simulink model "MIL4L3_SW6_V1_20220211"  (R2018b)
settings: Solver=FixedStepAuto  StartTime=0.0  StopTime=inf  FixedStep=0.001  RelTol=1e-3
PreLoadFcn:
  | A0_MILtest;
undefined symbols (not defined in the file or in its folder): Clb_ICADirect_LaneDisp_StateFive, Clb_ICADirect_LaneDisp_StateFour, Clb_ICADirect_LaneDisp_StateOne, Clb_ICADirect_LaneDisp_StateThree, Clb_ICADirect_LaneDisp_StateTwo, Clb_ICADirect_LaneDisp_StateZero, Clb_ICADirect_LaneDispSW, Clb_ICADirect_TrnLghtsCom_Switch, Clb_ICADirect_TrnLghtsCom_Value, Clb_ICADirect_TrnLghtsCrtl_Inhb, IMAP_Clb_ACU_Driver_Belt, IMAP_Clb_ACU_Driver_Belt_Over, IMAP_Clb_ACU_Passenger_Belt, IMAP_Clb_ACU_Passenger_Belt_Over, IMAP_Clb_ACU_RearLeft_Belt, IMAP_Clb_ACU_RearLeft_Belt_Over, IMAP_Clb_ACU_RearMiddle_Belt, IMAP_Clb_ACU_RearMiddle_Belt_Over, IMAP_Clb_ACU_RearRight_Belt, IMAP_Clb_ACU_RearRight_Belt_Over, IMAP_Clb_AEB_Switch, IMAP_Clb_AEB_Switch_Over, IMAP_Clb_ALC_TLC_Mode, IMAP_Clb_ALC_TLC_Mode_Over, IMAP_Clb_BCM_Battery_Voltage, IMAP_Clb_BCM_Battery_Voltage_Over, IMAP_Clb_BCM_BrakeLamp_State, IMAP_Clb_BCM_BrakeLamp_State_Over, IMAP_Clb_BCM_CHMSL_Status, IMAP_Clb_BCM_CHMSL_Status_Over, IMAP_Clb_BCM_Door_Lock_State, IMAP_Clb_BCM_Door_Lock_State_Over, IMAP_Clb_BCM_FrontWiper_State, IMAP_Clb_BCM_FrontWiper_State_Over, IMAP_Clb_BCM_FrontWiper_Switch, IMAP_Clb_BCM_FrontWiper_Switch_Over, IMAP_Clb_BCM_HazardLamp, IMAP_Clb_BCM_HazardLamp_Over, IMAP_Clb_BCM_HazardLamp_Switch, IMAP_Clb_BCM_HazardLamp_Switch_Over, IMAP_Clb_BCM_HighBeam_State, IMAP_Clb_BCM_HighBeam_State_Over, IMAP_Clb_BCM_Ignition_State, IMAP_Clb_BCM_Ignition_State_Over, IMAP_Clb_BCM_IHBC_Enabled, IMAP_Clb_BCM_IHBC_Enabled_Over, IMAP_Clb_BCM_Left_Light, IMAP_Clb_BCM_Left_Light_Over, IMAP_Clb_BCM_LeftTurn_Switch, IMAP_Clb_BCM_LeftTurn_Switch_Over, IMAP_Clb_BCM_LF_Door_State, IMAP_Clb_BCM_LF_Door_State_Over, IMAP_Clb_BCM_LowBeam_State, IMAP_Clb_BCM_LowBeam_State_Over, IMAP_Clb_BCM_LR_Door_State, IMAP_Clb_BCM_LR_Door_State_Over, IMAP_Clb_BCM_RF_Door_State, IMAP_Clb_BCM_RF_Door_State_Over, IMAP_Clb_BCM_Right_Light, IMAP_Clb_BCM_Right_Light_Over ... (+547)
libraries: CarMaker4SL x2153, simulink x292, dspstat3 x3, canmsglib x2, simulink_extras x1
(part 4 of 52)

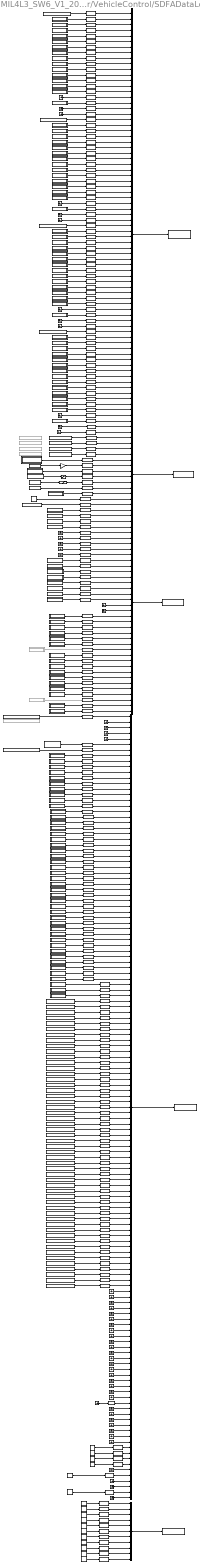
== system MIL4L3_SW6_V1_20220211/CarMaker/VehicleControl/SDFADataLog ==
  ACCEL_LONGI_CALIB2 : Saturate  UpperLimit=40.92  LowerLimit=-40.96
  BusCreator : BusCreator  Inputs=11
  BusCreator1 : BusCreator  Inputs=80
  BusCreator2 : BusCreator  Inputs=40
  BusCreator3 : BusCreator  Inputs=6
  BusCreator4 : BusCreator  Inputs=141
  CIPV_ID1 : Subsystem
  Constant{,1..3,8,10..21} (17 alike) : Constant  Value=0
  Constant9 : Constant
  Data Type  Conversion{1..3,6,508} (5 alike) : DataTypeConversion
  Data Type Conversion{,1..82,85,98,118,128..129,131..251,253..265,267,398,442..444,446..449,451..455} (236 alike) : DataTypeConversion
  Define CM Dict : CarMaker4SL/Define CM Dict  Commented=on  xname=User.IO.Out.CRFLstatus  xmono=off  xtype=Double4  xdvaplace=None  xnstates=0  xfirststate=0  xinitial=0
  Define CM Dict1 : CarMaker4SL/Define CM Dict  Commented=on  xname=User.IO.Out.CRFRstatus  xmono=off  xtype=Double4  xdvaplace=None  xnstates=0  xfirststate=0  xinitial=0
  Define CM Dict3 : CarMaker4SL/Define CM Dict  Commented=on  xname=User.IO.Out.CRRLstatus  xmono=off  xtype=Double4  xdvaplace=None  xnstates=0  xfirststate=0  xinitial=0
  Define CM Dict4 : CarMaker4SL/Define CM Dict  Commented=on  xname=User.IO.Out.CRRRstatus  xmono=off  xtype=Double4  xdvaplace=None  xnstates=0  xfirststate=0  xinitial=0
  Define CM Dict7 : CarMaker4SL/Define CM Dict  Commented=on  xname=User.IO.Out.IFCState  xmono=off  xtype=Double4  xdvaplace=IO_Out  xnstates=0  xfirststate=0  xinitial=9
  Gain10 : Gain  Gain=3.6
  Ground{,1..47,52,56..61} (55 alike) : Ground
  Lateral_acceleration1 : CarMaker4SL/Read CM Dict  xname=Car.ay  xsync=off
  Lateral_acceleration2 : CarMaker4SL/Read CM Dict  xname=User.IO.Out.CRFLstatus  xsync=off
  Lateral_acceleration3 : CarMaker4SL/Read CM Dict  xname=User.IO.Out.CRFRstatus  xsync=off
  Lateral_acceleration4 : CarMaker4SL/Read CM Dict  xname=User.IO.Out.CRRLstatus  xsync=off
  Lateral_acceleration5 : CarMaker4SL/Read CM Dict  xname=User.IO.Out.CRRRstatus  xsync=off
  Read CM Dict : CarMaker4SL/Read CM Dict  xname=User.IO.Out.IFC_Line01_CurvChange  xsync=off
  Read CM Dict1 : CarMaker4SL/Read CM Dict  xname=User.IO.Out.NumberOfObjects_S3  xsync=off
  Read CM Dict10 : CarMaker4SL/Read CM Dict  xname=User.IO.Out.IFC_Line01_Dy  xsync=off
  Read CM Dict11 : CarMaker4SL/Read CM Dict  xname=User.IO.Out.IFC_Line01_ExistProb  xsync=off
  Read CM Dict12 : CarMaker4SL/Read CM Dict  xname=User.IO.Out.IFC_Line01_MeasureType  xsync=off
  Read CM Dict13 : CarMaker4SL/Read CM Dict  xname=User.IO.Out.IFC_Line01_Type  xsync=off
  Read CM Dict14 : CarMaker4SL/Read CM Dict  xname=User.IO.Out.IFC_Line01_LineID  xsync=off
  Read CM Dict15 : CarMaker4SL/Read CM Dict  xname=User.IO.Out.IFC_Line01_TypeConf  xsync=off
  Read CM Dict16 : CarMaker4SL/Read CM Dict  xname=User.IO.Out.IFC_Line01_ColorClass  xsync=off
  Read CM Dict17 : CarMaker4SL/Read CM Dict  xname=User.IO.Out.IFC_Line01_DxStart  xsync=off
  Read CM Dict18 : CarMaker4SL/Read CM Dict  xname=User.IO.Out.IFC_Line01_DxEnd  xsync=off
  Read CM Dict19 : CarMaker4SL/Read CM Dict  xname=User.IO.Out.IFC_Line01_LineWidth  xsync=off
  Read CM Dict2 : CarMaker4SL/Read CM Dict  xname=User.IO.Out.IFCState  xsync=off
  Read CM Dict20 : CarMaker4SL/Read CM Dict  xname=User.IO.Out.IFC_Line02_CurvChange  xsync=off
  Read CM Dict21 : CarMaker4SL/Read CM Dict  xname=User.IO.Out.IFC_Line02_Curv  xsync=off
  Read CM Dict22 : CarMaker4SL/Read CM Dict  xname=User.IO.Out.IFC_Line02_HeadingAngle  xsync=off
  Read CM Dict23 : CarMaker4SL/Read CM Dict  xname=User.IO.Out.IFC_Line02_Dy  xsync=off
  Read CM Dict24 : CarMaker4SL/Read CM Dict  xname=User.IO.Out.IFC_Line02_ExistProb  xsync=off
  Read CM Dict25 : CarMaker4SL/Read CM Dict  xname=Car.ax  xsync=off
  Read CM Dict26 : CarMaker4SL/Read CM Dict  xname=Car.v  xsync=off
  Read CM Dict27 : CarMaker4SL/Read CM Dict  xname=Steer.WhlAng  xsync=off
  Read CM Dict28 : CarMaker4SL/Read CM Dict  xname=User.IO.Out.IFC_Line02_MeasureType  xsync=off
  Read CM Dict29 : CarMaker4SL/Read CM Dict  xname=User.IO.Out.IFC_Line02_Type  xsync=off
  Read CM Dict3 : CarMaker4SL/Read CM Dict  xname=User.IO.Out.NumberOfObjects_S0  xsync=off
  Read CM Dict30 : CarMaker4SL/Read CM Dict  xname=User.IO.Out.IFC_Line02_LineID  xsync=off
  Read CM Dict31 : CarMaker4SL/Read CM Dict  xname=User.IO.Out.IFC_Line02_TypeConf  xsync=off
  Read CM Dict32 : CarMaker4SL/Read CM Dict  xname=User.IO.Out.IFC_Line02_ColorClass  xsync=off
  Read CM Dict33 : CarMaker4SL/Read CM Dict  xname=User.IO.Out.IFC_Line02_DxStart  xsync=off
  Read CM Dict34 : CarMaker4SL/Read CM Dict  xname=User.IO.Out.IFC_Line02_DxEnd  xsync=off
  Read CM Dict35 : CarMaker4SL/Read CM Dict  xname=User.IO.Out.IFC_Line02_LineWidth  xsync=off
  Read CM Dict36 : CarMaker4SL/Read CM Dict  xname=User.IO.Out.IFC_Line03_CurvChange  xsync=off
  Read CM Dict37 : CarMaker4SL/Read CM Dict  xname=User.IO.Out.IFC_Line03_Curv  xsync=off
  Read CM Dict38 : CarMaker4SL/Read CM Dict  xname=User.IO.Out.IFC_Line03_HeadingAngle  xsync=off
  Read CM Dict39 : CarMaker4SL/Read CM Dict  xname=User.IO.Out.IFC_Line03_Dy  xsync=off
  Read CM Dict4 : CarMaker4SL/Read CM Dict  xname=User.IO.Out.NumberOfObjects_S1  xsync=off
  Read CM Dict40 : CarMaker4SL/Read CM Dict  xname=User.IO.Out.IFC_Line03_ExistProb  xsync=off
  Read CM Dict41 : CarMaker4SL/Read CM Dict  xname=User.IO.Out.IFC_Line03_MeasureType  xsync=off
  Read CM Dict42 : CarMaker4SL/Read CM Dict  xname=User.IO.Out.IFC_Line03_Type  xsync=off
  Read CM Dict43 : CarMaker4SL/Read CM Dict  xname=User.IO.Out.IFC_Line03_LineID  xsync=off
  Read CM Dict44 : CarMaker4SL/Read CM Dict  xname=User.IO.Out.IFC_Line03_TypeConf  xsync=off
  Read CM Dict45 : CarMaker4SL/Read CM Dict  xname=User.IO.Out.IFC_Line03_ColorClass  xsync=off
  Read CM Dict46 : CarMaker4SL/Read CM Dict  xname=User.IO.Out.IFC_Line03_DxStart  xsync=off
  Read CM Dict47 : CarMaker4SL/Read CM Dict  xname=User.IO.Out.IFC_Line03_DxEnd  xsync=off
  Read CM Dict48 : CarMaker4SL/Read CM Dict  xname=User.IO.Out.IFC_Line03_LineWidth  xsync=off
  Read CM Dict49 : CarMaker4SL/Read CM Dict  xname=User.IO.Out.IFC_Line04_CurvChange  xsync=off
  Read CM Dict5 : CarMaker4SL/Read CM Dict  xname=User.IO.Out.NumberOfObjects_S2  xsync=off
  Read CM Dict50 : CarMaker4SL/Read CM Dict  xname=User.IO.Out.IFC_Line04_Curv  xsync=off
  Read CM Dict51 : CarMaker4SL/Read CM Dict  xname=User.IO.Out.IFC_Line04_HeadingAngle  xsync=off
  Read CM Dict52 : CarMaker4SL/Read CM Dict  xname=User.IO.Out.IFC_Line04_Dy  xsync=off
  Read CM Dict53 : CarMaker4SL/Read CM Dict  xname=User.IO.Out.IFC_Line04_ExistProb  xsync=off
  Read CM Dict54 : CarMaker4SL/Read CM Dict  xname=User.IO.Out.IFC_Line04_MeasureType  xsync=off
  Read CM Dict55 : CarMaker4SL/Read CM Dict  xname=User.IO.Out.IFC_Line04_Type  xsync=off
  Read CM Dict56 : CarMaker4SL/Read CM Dict  xname=User.IO.Out.IFC_Line04_LineID  xsync=off
  Read CM Dict57 : CarMaker4SL/Read CM Dict  xname=User.IO.Out.IFC_Line04_TypeConf  xsync=off
  Read CM Dict58 : CarMaker4SL/Read CM Dict  xname=User.IO.Out.IFC_Line04_ColorClass  xsync=off
  Read CM Dict59 : CarMaker4SL/Read CM Dict  xname=User.IO.Out.IFC_Line04_DxStart  xsync=off
  Read CM Dict6 : CarMaker4SL/Read CM Dict  xname=User.IO.Out.NumberOfObj  xsync=off
  Read CM Dict60 : CarMaker4SL/Read CM Dict  xname=User.IO.Out.IFC_Line04_DxEnd  xsync=off
  Read CM Dict61 : CarMaker4SL/Read CM Dict  xname=User.IO.Out.IFC_Line04_LineWidth  xsync=off
  Read CM Dict62 : CarMaker4SL/Read CM Dict  xname=User.IO.Out.ObjCount  xsync=off
  Read CM Dict8 : CarMaker4SL/Read CM Dict  xname=User.IO.Out.IFC_Line01_Curv  xsync=off
  Read CM Dict9 : CarMaker4SL/Read CM Dict  xname=User.IO.Out.IFC_Line01_HeadingAngle  xsync=off
  Saturation3 : Saturate  UpperLimit=780  LowerLimit=-780
  Subsystem : Subsystem
  Subsystem1 : Subsystem
  Subsystem10 : Subsystem
  Subsystem100 : Subsystem
  Subsystem103 : Subsystem
  Subsystem107 : Subsystem
  Subsystem108 : Subsystem
  Subsystem109 : Subsystem
  Subsystem11 : Subsystem
  Subsystem110 : Subsystem
  Subsystem111 : Subsystem
  Subsystem112 : Subsystem
  Subsystem113 : Subsystem
  Subsystem114 : Subsystem
  Subsystem115 : Subsystem
  Subsystem116 : Subsystem
  Subsystem117 : Subsystem
  Subsystem118 : Subsystem
  Subsystem119 : Subsystem
  Subsystem12 : Subsystem
  Subsystem120 : Subsystem
  Subsystem13 : Subsystem  Commented=on
  Subsystem14 : Subsystem
  Subsystem149 : Subsystem
  Subsystem150 : Subsystem
  Subsystem160 : Subsystem
  Subsystem171 : Subsystem
  Subsystem174 : Subsystem
  Subsystem175 : Subsystem
  Subsystem176 : Subsystem
  Subsystem177 : Subsystem
  Subsystem178 : Subsystem
  Subsystem179 : Subsystem
  Subsystem180 : Subsystem
  Subsystem181 : Subsystem
  Subsystem182 : Subsystem
  Subsystem183 : Subsystem
  Subsystem184 : Subsystem
  Subsystem185 : Subsystem
  Subsystem186 : Subsystem
  Subsystem187 : Subsystem
  Subsystem188 : Subsystem
  Subsystem189 : Subsystem
  Subsystem190 : Subsystem
  Subsystem191 : Subsystem
  Subsystem192 : Subsystem
  Subsystem193 : Subsystem
  Subsystem194 : Subsystem
  Subsystem195 : Subsystem
  Subsystem196 : Subsystem
  Subsystem197 : Subsystem
  Subsystem198 : Subsystem
  Subsystem199 : Subsystem
  Subsystem2 : Subsystem
  Subsystem20 : Subsystem
  Subsystem200 : Subsystem
  Subsystem201 : Subsystem
  Subsystem202 : Subsystem
  Subsystem203 : Subsystem
  Subsystem204 : Subsystem
  Subsystem205 : Subsystem
  Subsystem206 : Subsystem
  Subsystem208 : Subsystem
  Subsystem209 : Subsystem
  Subsystem210 : Subsystem
  Subsystem211 : Subsystem
  Subsystem212 : Subsystem
  Subsystem213 : Subsystem  Commented=on
  Subsystem214 : Subsystem
  Subsystem215 : Subsystem
  Subsystem216 : Subsystem
  Subsystem217 : Subsystem
  Subsystem218 : Subsystem
  Subsystem219 : Subsystem
  Subsystem220 : Subsystem
  Subsystem221 : Subsystem
  Subsystem222 : Subsystem
  Subsystem223 : Subsystem
  Subsystem224 : Subsystem
  Subsystem225 : Subsystem
  Subsystem226 : Subsystem
  Subsystem227 : Subsystem
  Subsystem228 : Subsystem
  Subsystem232 : Subsystem
  Subsystem255 : Subsystem
  Subsystem283 : Subsystem
  Subsystem3 : Subsystem
  Subsystem40 : Subsystem
  Subsystem46 : Subsystem
  Subsystem47 : Subsystem
  Subsystem48 : Subsystem
  Subsystem49 : Subsystem
  Subsystem5 : Subsystem
  Subsystem50 : Subsystem
  Subsystem51 : Subsystem
  Subsystem52 : Subsystem
  Subsystem53 : Subsystem
  Subsystem54 : Subsystem
  Subsystem55 : Subsystem
  Subsystem56 : Subsystem
  Subsystem57 : Subsystem
  Subsystem58 : Subsystem
  Subsystem59 : Subsystem
  Subsystem6 : Subsystem
  Subsystem61 : Subsystem
  Subsystem66 : Subsystem
  Subsystem67 : Subsystem
  Subsystem68 : Subsystem
  Subsystem69 : Subsystem
  Subsystem7 : Subsystem
  Subsystem70 : Subsystem
  Subsystem71 : Subsystem
  Subsystem72 : Subsystem
  Subsystem73 : Subsystem
  Subsystem74 : Subsystem
  Subsystem75 : Subsystem
  Subsystem76 : Subsystem
  Subsystem77 : Subsystem
  Subsystem78 : Subsystem
  Subsystem79 : Subsystem
  Subsystem8 : Subsystem
  Subsystem81 : Subsystem
  Subsystem85 : Subsystem
  Subsystem86 : Subsystem
  Subsystem87 : Subsystem
  Subsystem88 : Subsystem
  Subsystem89 : Subsystem
  Subsystem9 : Subsystem
  Subsystem90 : Subsystem
  Subsystem91 : Subsystem
  Subsystem92 : Subsystem
  Subsystem93 : Subsystem
  Subsystem94 : Subsystem
  Subsystem95 : Subsystem
  Subsystem96 : Subsystem
  Subsystem97 : Subsystem
  Subsystem98 : Subsystem
  To Workspace : ToWorkspace  VariableName=CameraDataLog  SaveFormat=Timeseries  SampleTime=-1
  To Workspace1 : ToWorkspace  VariableName=RadarDataLog  SaveFormat=Timeseries  SampleTime=-1
  To Workspace2 : ToWorkspace  VariableName=VehicleDataLog  SaveFormat=Timeseries  SampleTime=-1
  To Workspace3 : ToWorkspace  VariableName=CRDataLog  SaveFormat=Timeseries  SampleTime=-1
  To Workspace4 : ToWorkspace  VariableName=LAPDataLog  SaveFormat=Timeseries  SampleTime=-1
  wires:
  BusCreator3/1 -> To Workspace2/1  "VehicleData"
  BusCreator4/1 -> To Workspace/1  "CameraData"
  BusCreator2/1 -> To Workspace1/1  "RadarData"
  BusCreator1/1 -> To Workspace3/1  "CRData"
  Subsystem13/1(BrakingAllowed) -> Data Type Conversion82/1
  Data Type Conversion232/1 -> BusCreator4/86  "LH_Lanemark_Type_Conf_03"
  Subsystem6/1(obj_HeadOrientation) -> Data Type Conversion74/1
  Data Type Conversion70/1 -> BusCreator2/32  "ObjectAge"
  Data Type Conversion/1 -> BusCreator4/132  "CorrCoeff_x_vx"
  Data Type Conversion215/1 -> BusCreator4/70  "IFC_Line02_MeasureType"
  Data Type Conversion27/1 -> BusCreator4/20  "IFC_obj_abs_AxStdDev"
  Data Type Conversion235/1 -> BusCreator4/12  "IFC_obj_VxValid"
  Data Type Conversion249/1 -> BusCreator4/101  "IFC_Line04_DxStart"
  Data Type Conversion59/1 -> BusCreator4/57  "IFC_Line01_MeasureType"
  Read CM Dict34/1 -> Data Type Conversion221/1
  Read CM Dict36/1 -> Data Type Conversion223/1
  Subsystem10/1(obj_PhiBottom) -> Data Type Conversion78/1
  Subsystem7/1(obj_DirIndicator) -> Data Type Conversion75/1
  Data Type Conversion261/1 -> BusCreator2/9  "RelativeLongVelo"
  Subsystem198/1(obj_Rel_VxSTD) -> Data Type Conversion29/1
  Data Type Conversion58/1 -> BusCreator4/56  "IFC_Line01_ExistProb"
  Data Type Conversion260/1 -> BusCreator2/10  "RelativeLatVelo"
  Data Type Conversion57/1 -> BusCreator4/55  "IFC_Line01_Dy"
  Data Type Conversion213/1 -> BusCreator4/8  "IFC_obj_ExistProb"
  Data Type Conversion197/1 -> BusCreator1/63  "RBtar_Yvelocity"
  Data Type Conversion74/1 -> BusCreator4/47  "IFC_obj_HeadOrientation"
  Subsystem191/1(obj_PhiBottomSTD) -> Data Type Conversion22/1
  Data Type Conversion51/1 -> BusCreator4/49  "IFC_obj_TTIPC"
  Data Type Conversion205/1 -> BusCreator1/70  "RBtar_Class"
  Read CM Dict10/1 -> Data Type Conversion57/1
  Gain10/1 -> Data Type  Conversion508/1  "Vehicle_speed_of_wheelsensor"
  Subsystem193/1(obj_DxSTD) -> Data Type Conversion24/1
  Read CM Dict48/1 -> Data Type Conversion237/1
  Data Type Conversion150/1 -> BusCreator1/13  "LFtar_Class"
  Subsystem20/1(Yaw_speed) -> Data Type  Conversion1/1  "Yaw_speed"
  Ground/1 -> BusCreator4/136  "IsNew"
  Subsystem180/1(WidhSTD) -> Data Type Conversion11/1
  Constant1/1 -> Data Type Conversion118/1
  Data Type Conversion129/1 -> BusCreator4/135  "CorrCoeff_x_vy"
  Data Type Conversion224/1 -> BusCreator4/11  "IFC_obj_Rel_Vx"
  Subsystem216/1(obj_Width) -> Data Type Conversion44/1
  Data Type Conversion194/1 -> BusCreator1/60  "RBtar_Xpos"
  Data Type Conversion195/1 -> BusCreator1/62  "RBtar_Xvelocity"
  Read CM Dict47/1 -> Data Type Conversion236/1
  Data Type Conversion53/1 -> BusCreator4/52  "IFC_Line01_CurvChange"
  Data Type Conversion151/1 -> BusCreator1/14  "LFtar_ReferencePoint"
  Data Type Conversion247/1 -> BusCreator4/99  "LH_Lanemark_Type_Conf_04"
  Read CM Dict26/1 -> Gain10/1
  Subsystem196/1(obj_abs_AxSTD) -> Data Type Conversion27/1
  Data Type Conversion118/1 -> BusCreator4/133  "CorrCoeff_y_vy"
  Constant/1 -> Data Type Conversion/1
  Data Type  Conversion1/1 -> BusCreator3/3  "SWINve_g_ESC_YawRate"
  Read CM Dict20/1 -> Data Type Conversion67/1
  Subsystem9/1(obj_angle_3D) -> Data Type Conversion77/1
  Data Type Conversion65/1 -> BusCreator4/63  "IFC_Line01_DxEnd"
  Read CM Dict53/1 -> Data Type Conversion242/1
  Read CM Dict18/1 -> Data Type Conversion65/1
  Read CM Dict46/1 -> Data Type Conversion234/1
  Read CM Dict60/1 -> Data Type Conversion250/1
  Subsystem201/1(AbsoluteLatAcc) -> Data Type Conversion255/1
  Data Type Conversion30/1 -> BusCreator4/17  "IFC_obj_Rel_VyStdDev"
  Ground34/1 -> BusCreator4/127  "FS_Blur_Image_0"
  Subsystem150/1(AbsoluteLongAcc) -> Data Type Conversion258/1
  Subsystem199/1(obj_Rel_VySTD) -> Data Type Conversion30/1
  Subsystem204/1(obj_abs_Ay) -> Data Type Conversion33/1
  Ground52/1 -> Data Type Conversion72/1
  Data Type Conversion241/1 -> BusCreator4/94  "IFC_Line04_Dy"
  Data Type Conversion254/1 -> BusCreator2/23  "ClassType"
  Subsystem228/1(obj_Type) -> Data Type Conversion50/1
  Subsystem78/1(RFtar_ReferencePoint) -> Data Type Conversion168/1  "RFtar_ReferencePoint"
  Ground25/1 -> BusCreator4/123  "IFC_Roaddge02_LineID"
  Data Type Conversion147/1 -> BusCreator1/10  "LFtar_Length"
  Data Type Conversion85/1 -> BusCreator3/1  "system_clock"
  Data Type Conversion133/1 -> BusCreator1/79
  Read CM Dict28/1 -> Data Type Conversion215/1
  Data Type  Conversion6/1 -> BusCreator3/5  "SWINve_g_ESC_LongitudinalAccelaration"
  Subsystem227/1(obj_Measured) -> Data Type Conversion52/1
  Data Type Conversion239/1 -> BusCreator4/92  "IFC_Line04_Curv"
  Subsystem160/1(obj_Rel_Vx) -> Data Type Conversion224/1
  Read CM Dict43/1 -> Data Type Conversion231/1
  Subsystem195/1(obj_PhiLeftSTD) -> Data Type Conversion26/1
  Data Type Conversion5/1 -> BusCreator2/7  "LateralDistanceSTD"
  Read CM Dict32/1 -> Data Type Conversion219/1
  Read CM Dict27/1 -> Saturation3/1  "Steering_wheel_angle"
  Subsystem232/1(ClassProbValue) -> Data Type Conversion253/1
  Data Type Conversion75/1 -> BusCreator4/44  "IFC_obj_DirIndicator"
  Read CM Dict42/1 -> Data Type Conversion230/1
  Data Type  Conversion2/1 -> BusCreator3/4  "SWINve_g_SAS_SteeringAngle"
  Ground3/1 -> Data Type Conversion261/1
  Subsystem76/1(RFtar_ExistenceProbability) -> Data Type Conversion166/1  "RFtar_ExistenceProbability"
  Subsystem174/1(LateralDistanceSTD) -> Data Type Conversion5/1
  Subsystem118/1(RBtar_Class) -> Data Type Conversion205/1  "RBtar_Class"
  Read CM Dict35/1 -> Data Type Conversion222/1
  Ground39/1 -> BusCreator4/131  "FS_Out_Of_Focus_0"
  Data Type Conversion220/1 -> BusCreator4/75  "IFC_Line02_DxStart"
  Read CM Dict23/1 -> Data Type Conversion212/1
  Ground57/1 -> BusCreator4/3  "FS_Sun_Ray_0"
  Data Type Conversion227/1 -> BusCreator4/81  "IFC_Line03_Dy"
  Read CM Dict33/1 -> Data Type Conversion220/1
  Subsystem175/1(LongDistanceSTD) -> Data Type Conversion4/1
  Subsystem52/1(LFtar_Yacceleration) -> Data Type Conversion145/1  "LFtar_Yacceleration"
  Ground9/1 -> Data Type Conversion263/1
  Subsystem213/1(Height) -> Data Type Conversion42/1
  Subsystem176/1(AbsoluteLongAccSTD) -> Data Type Conversion7/1
  Data Type Conversion18/1 -> BusCreator4/40  "IFC_obj_HeightStdDev"
  Ground61/1 -> BusCreator2/22  "AbsAccCov"
  Data Type Conversion221/1 -> BusCreator4/76  "IFC_Line02_DxEnd"
  Subsystem149/1(obj_ExistProb) -> Data Type Conversion213/1
  Subsystem219/1(YawAngle) -> Data Type Conversion36/1
  Data Type Conversion258/1 -> BusCreator2/15  "AbsoluteLongAcc"
  Data Type Conversion46/1 -> BusCreator2/25  "Length"
  Subsystem1/1(LongDistance) -> Data Type Conversion267/1
  Read CM Dict59/1 -> Data Type Conversion249/1
  Data Type Conversion211/1 -> BusCreator4/67  "IFC_Line02_HeadingAngle"
  Data Type Conversion226/1 -> BusCreator4/80  "IFC_Line03_HeadingAngle"
  Data Type Conversion257/1 -> BusCreator2/40  "ExistenceProb"
  Read CM Dict9/1 -> Data Type Conversion55/1
  Subsystem107/1(RBtar_id) -> Data Type Conversion192/1  "RBtar_id"
  Subsystem221/1(MovementStatus) -> Data Type Conversion34/1
  Data Type Conversion216/1 -> BusCreator4/71  "IFC_Line02_Type"
  Read CM Dict52/1 -> Data Type Conversion241/1
  Data Type Conversion8/1 -> BusCreator2/18  "AbsLatVeloSTD"
  Read CM Dict13/1 -> Data Type Conversion61/1
  Data Type Conversion12/1 -> BusCreator2/30  "HeightSTD"
  Read CM Dict58/1 -> Data Type Conversion248/1
  Read CM Dict50/1 -> Data Type Conversion239/1
  Subsystem189/1(obj_HeadingSTD) -> Data Type Conversion20/1
  Subsystem209/1(Length) -> Data Type Conversion46/1
  Subsystem66/1(RFtar_id) -> Data Type Conversion154/1  "RFtar_id"
  Data Type Conversion33/1 -> BusCreator4/21  "IFC_obj_abs_Ay"
  Subsystem90/1(LBtar_Xacceleration) -> Data Type Conversion179/1  "LBtar_Xacceleration"
  Read CM Dict16/1 -> Data Type Conversion63/1
  Data Type Conversion191/1 -> BusCreator1/58  "RBtar_number"
  Read CM Dict17/1 -> Data Type Conversion64/1
  Data Type Conversion217/1 -> BusCreator4/72  "IFC_Line02_LineID"
  Data Type Conversion24/1 -> BusCreator4/24  "IFC_obj_DxStdDev"
  Data Type  Conversion3/1 -> BusCreator3/6  "SWINve_g_ESC_LateralAccelaration"
  Subsystem192/1(obj_Rel_Vy) -> Data Type Conversion246/1
  Ground18/1 -> Data Type Conversion206/1  "RBtar_ObjectInfo"
  Ground31/1 -> BusCreator4/117  "IFC_Roaddge02_Curv"
  Read CM Dict57/1 -> Data Type Conversion247/1
  Subsystem222/1(MeasurementStatus) -> Data Type Conversion32/1
  Data Type Conversion264/1 -> BusCreator2/3  "NumberOfObj"
  Read CM Dict3/1 -> Data Type Conversion172/1  "LBtar_number"
  ACCEL_LONGI_CALIB2/1 -> Data Type  Conversion6/1  "ACCEL_LONGI_CALIB"
  Subsystem203/1(obj_abs_Ax) -> Data Type Conversion23/1
  Read CM Dict45/1 -> Data Type Conversion233/1
  Data Type Conversion253/1 -> BusCreator2/24  "ClassProbValue"
  Data Type Conversion156/1 -> BusCreator1/23  "RFtar_Ypos"
  Data Type Conversion256/1 -> BusCreator2/17  "AbsoluteLatVelo"
  Subsystem214/1(obj_PhiRight) -> Data Type Conversion41/1
  Data Type Conversion52/1 -> BusCreator4/51  "IFC_obj_Measured"
  Ground26/1 -> BusCreator4/113  "IFC_Roaddge01_LineID"
  Data Type Conversion66/1 -> BusCreator4/64  "IFC_Line01_LineWidth"
  Subsystem255/1(AbsoluteLongVeloSTD) -> Data Type Conversion6/1
  Subsystem55/1(LFtar_Orientation) -> Data Type Conversion148/1  "LFtar_Orientation"
  Read CM Dict8/1 -> Data Type Conversion54/1
  Data Type Conversion42/1 -> BusCreator2/29  "Height"
  Data Type Conversion16/1 -> BusCreator4/38  "IFC_obj_WidthStdDev"
  Data Type Conversion20/1 -> BusCreator4/46  "IFC_obj_HeadingStdDev"
  Data Type Conversion233/1 -> BusCreator4/87  "IFC_Line03_ColorClass"
  Data Type Conversion225/1 -> BusCreator4/79  "IFC_Line03_Curv"
  Data Type Conversion41/1 -> BusCreator4/29  "IFC_obj_PhiRight"
  Data Type Conversion63/1 -> BusCreator4/61  "IFC_Line01_ColorClass"
  Ground58/1 -> BusCreator4/4  "FS_Fog"
  Data Type Conversion37/1 -> BusCreator4/25  "IFC_obj_Dy"
  Ground17/1 -> Data Type Conversion152/1  "LFtar_timestamp"
  Subsystem119/1(RBtar_ReferencePoint) -> Data Type Conversion204/1  "RBtar_ReferencePoint"
  Data Type Conversion243/1 -> BusCreator4/96  "IFC_Line04_MeasureType"
  Data Type Conversion49/1 -> BusCreator4/45  "IFC_obj_Heading"
  Data Type Conversion265/1 -> BusCreator2/2  "ObjectListQuali"
  Data Type Conversion55/1 -> BusCreator4/54  "IFC_Line01_HeadingAngle"
  Data Type Conversion40/1 -> BusCreator2/31  "ObjectID"
  Subsystem177/1(AbsoluteLatVeloSTD) -> Data Type Conversion8/1
  Read CM Dict39/1 -> Data Type Conversion227/1
  Subsystem188/1(obj_LengthSTD) -> Data Type Conversion19/1
  Subsystem200/1(obj_abgle_3DSTD) -> Data Type Conversion31/1
  Saturation3/1 -> Data Type  Conversion2/1
  Data Type Conversion76/1 -> BusCreator4/35  "IFC_obj_angle_rate"
  Ground38/1 -> Data Type Conversion169/1  "RFtar_ObjectInfo"
  Data Type Conversion244/1 -> BusCreator4/97  "IFC_Line04_Type"
  Data Type Conversion248/1 -> BusCreator4/100  "IFC_Line04_ColorClass"
  Data Type Conversion29/1 -> BusCreator4/15  "IFC_obj_Rel_VxStdDev"
  Ground40/1 -> Data Type Conversion171/1  "RFtar_timestamp"
  Read CM Dict11/1 -> Data Type Conversion58/1
  Subsystem187/1(obj_HeightSTD) -> Data Type Conversion18/1
  Data Type Conversion10/1 -> BusCreator2/26  "LengthSTD"
  Ground28/1 -> BusCreator4/115  "IFC_Roaddge02_MessureType"
  Subsystem205/1(ClassType) -> Data Type Conversion254/1
  Read CM Dict5/1 -> Data Type Conversion138/1
  Data Type  Conversion508/1 -> BusCreator3/2  "SWINve_g_ESC_VeSpd"
  Subsystem224/1(obj_Heading) -> Data Type Conversion49/1
  Data Type Conversion1/1 -> BusCreator4/9  "IFC_obj_TypePron"
  Data Type Conversion181/1 -> BusCreator1/47  "LBtar_Width"
  Lateral_acceleration2/1 -> Data Type Conversion131/1
  Data Type Conversion155/1 -> BusCreator1/22  "RFtar_Xpos"
  Data Type Conversion171/1 -> BusCreator1/38  "RFtar_timestamp"
  Subsystem212/1(obj_PhiLeft) -> Data Type Conversion38/1
  Data Type Conversion79/1 -> BusCreator4/18  "IFC_obj_Rel_VyStdDevValid"
  Data Type Conversion21/1 -> BusCreator4/50  "IFC_obj_TTIPC_StdDev"
  Data Type Conversion238/1 -> BusCreator4/91  "IFC_Line04_CurvChange"
  Ground10/1 -> BusCreator4/108  "IFC_Roaddge01_HeadingAngle"
  Data Type Conversion31/1 -> BusCreator4/34  "IFC_obj_angle_3DStdDev"
  Ground56/1 -> BusCreator4/2  "FS_Low_Sun_0"
  Subsystem49/1(LFtar_Xvelocity) -> Data Type Conversion142/1  "LFtar_Xvelocity"
  Subsystem85/1(LBtar_id) -> Data Type Conversion173/1  "LBtar_id"
  Subsystem215/1(ObjectID) -> Data Type Conversion40/1
  Subsystem182/1(AbsoluteLatVelo) -> Data Type Conversion256/1
  Data Type Conversion7/1 -> BusCreator2/16  "AbsoluteLongAccSTD"
  Data Type Conversion28/1 -> BusCreator4/22  "IFC_obj_abs_AyStdDev"
  Read CM Dict15/1 -> Data Type Conversion62/1
  Subsystem202/1(obj_Rel_VyValid) -> Data Type Conversion2/1
  Data Type Conversion14/1 -> BusCreator2/35  "YawSTD"
  Data Type Conversion15/1 -> BusCreator4/30  "IFC_obj_PhiRightStdDev"
  Read CM Dict25/1 -> ACCEL_LONGI_CALIB2/1
  Data Type Conversion3/1 -> BusCreator2/6  "LatDistance"
  Ground21/1 -> BusCreator4/119  "IFC_Roaddge02_Dy"
  Read CM Dict21/1 -> Data Type Conversion68/1
  Read CM Dict38/1 -> Data Type Conversion226/1
  CIPV_ID1/1(Out1) -> Data Type Conversion39/1  "CIVP_ID"
  Ground19/1 -> BusCreator4/118  "IFC_Roaddge02_HeadingAngle"
  Data Type Conversion22/1 -> BusCreator4/32  "IFC_obj_PhiBottomStdDev"
  Data Type Conversion36/1 -> BusCreator2/34  "YawAngle"
  Ground16/1 -> BusCreator4/112  "IFC_Roaddge01_ExistProb"
  Data Type Conversion35/1 -> BusCreator4/23  "IFC_obj_Dx"
  Constant2/1 -> Data Type Conversion128/1
  Data Type Conversion186/1 -> BusCreator1/51  "LBtar_Class"
  Data Type Conversion43/1 -> BusCreator2/27  "Widh"
  Data Type Conversion38/1 -> BusCreator4/27  "IFC_obj_PhiLeft"
  Ground27/1 -> BusCreator4/114  "IFC_Roaddge02_Type"
  Data Type Conversion34/1 -> BusCreator2/36  "MovementStatus"
  Read CM Dict30/1 -> Data Type Conversion217/1
  Ground24/1 -> BusCreator4/121  "IFC_Roaddge02_DxStart"
  Ground30/1 -> BusCreator4/116  "IFC_Roaddge02_CurvChange"
  Ground2/1 -> BusCreator4/122  "IFC_Roaddge02_ExistProb"
  Data Type Conversion219/1 -> BusCreator4/74  "IFC_Line02_ColorClass"
  Data Type Conversion78/1 -> BusCreator4/31  "IFC_obj_PhiBottom"
  Subsystem184/1(obj_PhiRightSTD) -> Data Type Conversion15/1
  Data Type Conversion230/1 -> BusCreator4/84  "IFC_Line03_Type"
  Subsystem11/1(obj_Rel_VyStdDevValid) -> Data Type Conversion79/1
  Ground33/1 -> BusCreator4/126  "FS_Splashes_0"
  Ground7/1 -> BusCreator4/107  "IFC_Roaddge01_Curv"
  Data Type Conversion73/1 -> BusCreator4/48  "IFC_obj_BrakeLight"
  Read CM Dict19/1 -> Data Type Conversion66/1
  Ground23/1 -> BusCreator4/120  "IFC_Roaddge02_DxEnd"
  Read CM Dict61/1 -> Data Type Conversion251/1
  Subsystem12/1(obj_Rel_VxStdDevValid) -> Data Type Conversion80/1
  Subsystem97/1(LBtar_ReferencePoint) -> Data Type Conversion187/1  "LBtar_ReferencePoint"
  Data Type Conversion11/1 -> BusCreator2/28  "WidhSTD"
  Ground14/1 -> Data Type Conversion158/1  "LFtar_ObjectInfo"
  Subsystem103/1(RBtar_ClassHighestProb) -> Data Type Conversion208/1  "RBtar_ClassHighestProb"
  Data Type Conversion141/1 -> BusCreator1/4  "LFtar_Ypos"
  Subsystem95/1(LBtar_ExistenceProbability) -> Data Type Conversion184/1  "LBtar_ExistenceProbability"
  Subsystem206/1(Latdistance) -> Data Type Conversion3/1
  Data Type Conversion61/1 -> BusCreator4/58  "IFC_Line01_Type"
  Read CM Dict40/1 -> Data Type Conversion228/1
  Data Type Conversion174/1 -> BusCreator1/18  "LFtar_MessageCounter"
  Data Type Conversion183/1 -> BusCreator1/49  "LBtar_Orientation"
  Subsystem57/1(LFtar_Class) -> Data Type Conversion150/1  "LFtar_Class"
  Subsystem120/1(RBtar_MovingState) -> Data Type Conversion136/1
  Data Type Conversion229/1 -> BusCreator4/83  "IFC_Line03_MeasureType"
  Subsystem54/1(LFtar_Length) -> Data Type Conversion147/1  "LFtar_Length"
  Ground15/1 -> Data Type Conversion174/1
  Subsystem194/1(obj_DySTD) -> Data Type Conversion25/1
  Ground37/1 -> BusCreator4/130  "FS_Full_Windshield_0"
  Subsystem59/1(LFtar_MovingState) -> Data Type Conversion185/1
  Data Type Conversion209/1 -> BusCreator1/76  "RBtar_timestamp"
  Subsystem111/1(RBtar_Yvelocity) -> Data Type Conversion197/1  "RBtar_Yvelocity"
  Subsystem77/1(RFtar_Class) -> Data Type Conversion167/1  "RFtar_Class"
  Data Type Conversion131/1 -> BusCreator1/77
  Subsystem88/1(LBtar_Xvelocity) -> Data Type Conversion177/1  "LBtar_Xvelocity"
  Read CM Dict37/1 -> Data Type Conversion225/1
  Ground22/1 -> Data Type Conversion188/1  "LBtar_ObjectInfo"
  Data Type Conversion67/1 -> BusCreator4/65  "IFC_Line02_CurvChange"
  Data Type Conversion132/1 -> BusCreator1/78
  Data Type Conversion64/1 -> BusCreator4/62  "IFC_Line01_DxStart"
  Subsystem115/1(RBtar_Length) -> Data Type Conversion201/1  "RBtar_Length"
  Subsystem81/1(RFtar_ClassHighestProb) -> Data Type Conversion170/1  "RFtar_ClassHighestProb"
  Data Type Conversion152/1 -> BusCreator1/19  "LFtar_timestamp"
  Subsystem108/1(RBtar_Xpos) -> Data Type Conversion194/1  "RBtar_Xpos"
  Subsystem114/1(RBtar_Width) -> Data Type Conversion199/1  "RBtar_Width"
  Data Type Conversion207/1 -> BusCreator1/37  "RFtar_MessageCounter"
  Subsystem110/1(RBtar_Xvelocity) -> Data Type Conversion195/1  "RBtar_Xvelocity"
  Subsystem113/1(RBtar_Yacceleration) -> Data Type Conversion200/1  "RBtar_Yacceleration"
  Read CM Dict44/1 -> Data Type Conversion232/1
  Subsystem72/1(RFtar_Yacceleration) -> Data Type Conversion162/1  "RFtar_Yacceleration"
  Data Type Conversion145/1 -> BusCreator1/8  "LFtar_Yacceleration"
  Ground45/1 -> Data Type Conversion135/1
  Subsystem50/1(LFtar_Yvelocity) -> Data Type Conversion143/1  "LFtar_Yvelocity"
  Data Type Conversion77/1 -> BusCreator4/33  "IFC_obj_angle_3D"
  Data Type Conversion153/1 -> BusCreator1/20  "RFtar_number"
  Data Type Conversion68/1 -> BusCreator4/66  "IFC_Line02_Curv"
  Data Type Conversion164/1 -> BusCreator1/29  "RFtar_Length"
  Ground41/1 -> Data Type Conversion207/1
  Subsystem58/1(LFtar_ReferencePoint) -> Data Type Conversion151/1  "LFtar_ReferencePoint"
  Subsystem96/1(LBtar_Class) -> Data Type Conversion186/1  "LBtar_Class"
  Data Type Conversion176/1 -> BusCreator1/42  "LBtar_Ypos"
  Data Type Conversion17/1 -> BusCreator4/36  "IFC_obj_angle_rate_StdDev"
  Subsystem87/1(LBtar_Ypos) -> Data Type Conversion176/1  "LBtar_Ypos"
  Subsystem69/1(RFtar_Xvelocity) -> Data Type Conversion157/1  "RFtar_Xvelocity"
  Data Type Conversion13/1 -> BusCreator4/1  "IFC_State"
  Subsystem74/1(RFtar_Length) -> Data Type Conversion164/1  "RFtar_Length"
  Subsystem100/1(LBtar_ClassHighestProb) -> Data Type Conversion189/1  "LBtar_ClassHighestProb"
  Subsystem68/1(RFtar_Ypos) -> Data Type Conversion156/1  "RFtar_Ypos"
  Data Type Conversion204/1 -> BusCreator1/71  "RBtar_ReferencePoint"
  Ground42/1 -> Data Type Conversion69/1
  Subsystem218/1(obj_Height) -> Data Type Conversion45/1
  Data Type Conversion201/1 -> BusCreator1/67  "RBtar_Length"
  Data Type Conversion136/1 -> BusCreator1/72  "RBtar_MovingState"
  Lateral_acceleration3/1 -> Data Type Conversion132/1
  Data Type Conversion246/1 -> BusCreator4/13  "IFC_obj_Rel_Vy"
  Subsystem94/1(LBtar_Orientation) -> Data Type Conversion183/1  "LBtar_Orientation"
  Subsystem283/1(AbsoluteLongVelo) -> Data Type Conversion262/1
  Subsystem92/1(LBtar_Width) -> Data Type Conversion181/1  "LBtar_Width"
  Data Type Conversion154/1 -> BusCreator1/21  "RFtar_id"
  Subsystem48/1(LFtar_Ypos) -> Data Type Conversion141/1  "LFtar_Ypos"
  Data Type Conversion210/1 -> BusCreator1/53  "LBtar_MovingState"
  Data Type Conversion47/1 -> BusCreator4/41  "IFC_obj_Length"
  Data Type Conversion135/1 -> BusCreator1/56  "LBtar_MessageCounter"
  Data Type Conversion157/1 -> BusCreator1/24  "RFtar_Xvelocity"
  Subsystem112/1(RBtar_Xacceleration) -> Data Type Conversion198/1  "RBtar_Xacceleration"
  Data Type Conversion198/1 -> BusCreator1/64  "RBtar_Xacceleration"
  Data Type Conversion162/1 -> BusCreator1/27  "RFtar_Yacceleration"
  Data Type Conversion137/1 -> BusCreator1/75  "RBtar_MessageCounter"
  Subsystem181/1(HeightSTD) -> Data Type Conversion12/1
  Read CM Dict6/1 -> Data Type Conversion264/1
  Subsystem75/1(RFtar_Orientation) -> Data Type Conversion165/1  "RFtar_Orientation"
  Data Type Conversion142/1 -> BusCreator1/5  "LFtar_Xvelocity"
  Data Type Conversion50/1 -> BusCreator4/10  "IFC_obj_Type"
  Ground59/1 -> BusCreator4/5  "FS_Rain"
  Subsystem210/1(obj_Dy) -> Data Type Conversion37/1
  Data Type Conversion192/1 -> BusCreator1/59  "RBtar_id"
  Data Type Conversion223/1 -> BusCreator4/78  "IFC_Line03_CurvChange"
  Data Type Conversion138/1 -> BusCreator1/1  "LFtar_number"
  Data Type Conversion56/1 -> BusCreator4/59  "IFC_Line01_LineID"
  Data Type Conversion160/1 -> BusCreator1/25  "RFtar_Yvelocity"
  Data Type Conversion158/1 -> BusCreator1/16  "LFtar_ObjectInfo"
  Ground46/1 -> Data Type Conversion137/1
  Data Type Conversion202/1 -> BusCreator1/68  "RBtar_Orientation"
  Subsystem179/1(LengthSTD) -> Data Type Conversion10/1
  Data Type Conversion189/1 -> BusCreator1/55  "LBtar_ClassHighestProb"
  Data Type Conversion182/1 -> BusCreator1/48  "LBtar_Length"
  Subsystem47/1(LFtar_Xpos) -> Data Type Conversion140/1  "LFtar_Xpos"
  Data Type Conversion146/1 -> BusCreator1/9  "LFtar_Width"
  Data Type Conversion184/1 -> BusCreator1/50  "LBtar_ExistenceProbability"
  Data Type Conversion143/1 -> BusCreator1/6  "LFtar_Yvelocity"
  Data Type Conversion193/1 -> BusCreator1/61  "RBtar_Ypos"
  Read CM Dict1/1 -> Data Type Conversion153/1  "RFtar_number"
  Data Type Conversion71/1 -> BusCreator2/33  "ReferencePoint"
  Subsystem3/1(ReferencePoint) -> Data Type Conversion71/1
  Data Type Conversion167/1 -> BusCreator1/32  "RFtar_Class"
  Data Type Conversion161/1 -> BusCreator1/26  "RFtar_Xacceleration"
  Data Type Conversion144/1 -> BusCreator1/7  "LFtar_Xacceleration"
  Data Type Conversion165/1 -> BusCreator1/30  "RFtar_Orientation"
  Data Type Conversion134/1 -> BusCreator1/80
  Data Type Conversion188/1 -> BusCreator1/54  "LBtar_ObjectInfo"
  Data Type Conversion170/1 -> BusCreator1/36  "RFtar_ClassHighestProb"
  Read CM Dict54/1 -> Data Type Conversion243/1
  Data Type Conversion250/1 -> BusCreator4/102  "IFC_Line04_DxEnd"
  Data Type Conversion179/1 -> BusCreator1/45  "LBtar_Xacceleration"
  Subsystem56/1(LFtar_ExistenceProbability) -> Data Type Conversion149/1  "LFtar_ExistenceProbability"
  Data Type Conversion163/1 -> BusCreator1/28  "RFtar_Width"
  Ground35/1 -> BusCreator4/128  "FS_Partical_Blockage_0"
  Lateral_acceleration5/1 -> Data Type Conversion134/1
  Ground32/1 -> BusCreator4/125  "FS_Out_Of_Calib"
  Data Type Conversion206/1 -> BusCreator1/73  "RBtar_ObjectInfo"
  Data Type Conversion200/1 -> BusCreator1/65  "RBtar_Yacceleration"
  Data Type Conversion166/1 -> BusCreator1/31  "RFtar_ExistenceProbability"
  Data Type Conversion149/1 -> BusCreator1/12  "LFtar_ExistenceProbability"
  Read CM Dict4/1 -> Data Type Conversion191/1  "RBtar_number"
  Subsystem98/1(LBtar_MovingState) -> Data Type Conversion210/1
  Lateral_acceleration4/1 -> Data Type Conversion133/1
  Data Type Conversion139/1 -> BusCreator1/2  "LFtar_id"
  Data Type Conversion203/1 -> BusCreator1/69  "RBtar_ExistenceProbability"
  Subsystem61/1(LFtar_ClassHighestProb) -> Data Type Conversion159/1  "LFtar_ClassHighestProb"
  Data Type Conversion98/1 -> BusCreator2/1  "TimeStamp"
  Data Type Conversion262/1 -> BusCreator2/13  "AbsoluteLongVelo"
  Constant3/1 -> Data Type Conversion129/1
  Subsystem211/1(Widh) -> Data Type Conversion43/1
  Data Type Conversion180/1 -> BusCreator1/46  "LBtar_Yacceleration"
  Subsystem217/1(obj_TypeProb) -> Data Type Conversion1/1
  Subsystem67/1(RFtar_Xpos) -> Data Type Conversion155/1  "RFtar_Xpos"
  Subsystem183/1(YawSTD) -> Data Type Conversion14/1
  Data Type Conversion60/1 -> BusCreator4/7  "IFC_ObjHdr_ObjCount"
  Subsystem225/1(ExistenceProb) -> Data Type Conversion257/1
  Data Type Conversion23/1 -> BusCreator4/19  "IFC_obj_abs_Ax"
  Data Type Conversion178/1 -> BusCreator1/44  "LBtar_Yvelocity"
  Ground20/1 -> Data Type Conversion209/1  "RBtar_timestamp"
  Subsystem197/1(obj_abs_AySTD) -> Data Type Conversion28/1
  Read CM Dict22/1 -> Data Type Conversion211/1
  Subsystem71/1(RFtar_Xacceleration) -> Data Type Conversion161/1  "RFtar_Xacceleration"
  Ground5/1 -> Data Type Conversion260/1
  Subsystem109/1(RBtar_Ypos) -> Data Type Conversion193/1  "RBtar_Ypos"
  Data Type Conversion128/1 -> BusCreator4/134  "CorrCoeff_y_vx"
  Subsystem223/1(obj_ID) -> Data Type Conversion48/1
  Data Type Conversion267/1 -> BusCreator2/4  "LongDistance"
  Subsystem226/1(obj_TTIPC) -> Data Type Conversion51/1
  Data Type Conversion44/1 -> BusCreator4/37  "IFC_obj_Width"
  Data Type Conversion234/1 -> BusCreator4/88  "IFC_Line03_DxStart"
  Subsystem186/1(obj_abgle_rate_STD) -> Data Type Conversion17/1
  Ground6/1 -> BusCreator4/106  "IFC_Roaddge01_CurvChange"
  Data Type Conversion148/1 -> BusCreator1/11  "LFtar_Orientation"
  Data Type Conversion218/1 -> BusCreator4/73  "LH_Lanemark_Type_Conf_02"
  Data Type Conversion208/1 -> BusCreator1/74  "RBtar_ClassHighestProb"
  Ground4/1 -> BusCreator4/105  "IFC_Roaddge01_MessureType"
  Data Type Conversion242/1 -> BusCreator4/95  "IFC_Line04_ExistProb"
  Subsystem53/1(LFtar_Width) -> Data Type Conversion146/1  "LFtar_Width"
  Data Type Conversion177/1 -> BusCreator1/43  "LBtar_Xvelocity"
  Data Type Conversion259/1 -> BusCreator2/11  "RelativeLatAcc"
  Data Type Conversion25/1 -> BusCreator4/26  "IFC_obj_DyStdDev"
  Subsystem171/1(obj_Rel_VxValid) -> Data Type Conversion235/1
  Data Type Conversion237/1 -> BusCreator4/90  "IFC_Line03_LineWidth"
  Data Type Conversion159/1 -> BusCreator1/17  "LFtar_ClassHighestProb"
  Ground13/1 -> BusCreator4/111  "IFC_Roaddge01_DxStart"
  Data Type Conversion173/1 -> BusCreator1/40  "LBtar_id"
  Subsystem117/1(RBtar_ExistenceProbability) -> Data Type Conversion203/1  "RBtar_ExistenceProbability"
  Subsystem116/1(RBtar_Orientation) -> Data Type Conversion202/1  "RBtar_Orientation"
  Read CM Dict62/1 -> Data Type Conversion60/1
  Data Type Conversion19/1 -> BusCreator4/42  "IFC_obj_LengthStdDev"
  Data Type Conversion175/1 -> BusCreator1/41  "LBtar_Xpos"
  Data Type Conversion212/1 -> BusCreator4/68  "IFC_Line02_Dy"
  Data Type Conversion80/1 -> BusCreator4/16  "IFC_obj_Rel_VxStdDevValid"
  Read CM Dict56/1 -> Data Type Conversion245/1
  Constant9/1 -> Data Type Conversion265/1
  Ground60/1 -> BusCreator2/21  "AbsVeloCov"
  Data Type Conversion82/1 -> BusCreator2/38  "BrakingAllowed"
  Read CM Dict55/1 -> Data Type Conversion244/1
  Ground29/1 -> Data Type Conversion190/1  "LBtar_timestamp"
  Subsystem14/1(RadarCrossSection) -> Data Type Conversion81/1
  Read CM Dict24/1 -> Data Type Conversion214/1
  Data Type Conversion222/1 -> BusCreator4/77  "IFC_Line02_LineWidth"
  Data Type Conversion39/1 -> BusCreator4/6  "IFC_VD_CIPV_ID"
  Subsystem/1(Out1) -> Data Type Conversion85/1
  Data Type Conversion2/1 -> BusCreator4/14  "IFC_obj_Rel_VyValid"
  Read CM Dict31/1 -> Data Type Conversion218/1
  Read CM Dict51/1 -> Data Type Conversion240/1
  Data Type Conversion4/1 -> BusCreator2/5  "LongDistanceSTD"
  Subsystem2/1(ObjectAge) -> Data Type Conversion70/1
  Data Type Conversion140/1 -> BusCreator1/3  "LFtar_Xpos"
  Lateral_acceleration1/1 -> Data Type  Conversion3/1  "Lateral_acceleration"
  Subsystem220/1(obj_Length) -> Data Type Conversion47/1
  Ground8/1 -> Data Type Conversion259/1
  Data Type Conversion26/1 -> BusCreator4/28  "IFC_obj_PhiLeftStdDev"
  Subsystem70/1(RFtar_Yvelocity) -> Data Type Conversion160/1  "RFtar_Yvelocity"
  Subsystem185/1(obj_WidthSTD) -> Data Type Conversion16/1
  Data Type Conversion172/1 -> BusCreator1/39  "LBtar_number"
  Subsystem89/1(LBtar_Yvelocity) -> Data Type Conversion178/1  "LBtar_Yvelocity"
  Data Type Conversion72/1 -> BusCreator2/8  "DistanceCovariance"
  Subsystem93/1(LBtar_Length) -> Data Type Conversion182/1  "LBtar_Length"
  Data Type Conversion240/1 -> BusCreator4/93  "IFC_Line04_HeadingAngle"
  Subsystem208/1(obj_Dx) -> Data Type Conversion35/1
  Subsystem190/1(obj_TTIPCSTD) -> Data Type Conversion21/1
  Read CM Dict2/1 -> Data Type Conversion13/1  "IFCState"
  Read CM Dict14/1 -> Data Type Conversion56/1
  Ground11/1 -> BusCreator4/109  "IFC_Roaddge01_Dy"
  Read CM Dict41/1 -> Data Type Conversion229/1
  Ground36/1 -> BusCreator4/129  "FS_Full_Blockage_0"
  Data Type Conversion190/1 -> BusCreator1/57  "LBtar_timestamp"
  Subsystem8/1(obj_angle_rate) -> Data Type Conversion76/1
  Subsystem5/1(obj_BrakeLight) -> Data Type Conversion73/1
  Data Type Conversion6/1 -> BusCreator2/14  "AbsLongVeloSTD"
  Data Type Conversion187/1 -> BusCreator1/52  "LBtar_ReferencePoint"
  Data Type Conversion9/1 -> BusCreator2/20  "AbsLatAccSTD"
  Data Type Conversion263/1 -> BusCreator2/12  "RelativeLongAcc"
  Data Type Conversion45/1 -> BusCreator4/39  "IFC_obj_Height"
  Ground1/1 -> BusCreator4/104  "IFC_Roaddge01_Type"
  Data Type Conversion236/1 -> BusCreator4/89  "IFC_Line03_DxEnd"
  Data Type Conversion169/1 -> BusCreator1/35  "RFtar_ObjectInfo"
  Read CM Dict49/1 -> Data Type Conversion238/1
  Subsystem46/1(LFtar_id) -> Data Type Conversion139/1  "LFtar_id"
  Data Type Conversion214/1 -> BusCreator4/69  "IFC_Line02_ExistProb"
  Data Type Conversion168/1 -> BusCreator1/33  "RFtar_ReferencePoint"
  Data Type Conversion199/1 -> BusCreator1/66  "RBtar_Width"
  Data Type Conversion62/1 -> BusCreator4/60  "LH_Lanemark_Type_Conf_01"
  Subsystem51/1(LFtar_Xacceleration) -> Data Type Conversion144/1  "LFtar_Xacceleration"
  Subsystem79/1(RFtar_MovingState) -> Data Type Conversion196/1
  Data Type Conversion32/1 -> BusCreator2/37  "MeasurementStatus"
  Data Type Conversion185/1 -> BusCreator1/15  "LFtar_MovingState"
  Subsystem91/1(LBtar_Yacceleration) -> Data Type Conversion180/1  "LBtar_Yacceleration"
  Subsystem40/1(TimeStamp) -> Data Type Conversion98/1
  Read CM Dict/1 -> Data Type Conversion53/1
  Subsystem178/1(AbsLatAccSTD) -> Data Type Conversion9/1
  Data Type Conversion48/1 -> BusCreator4/43  "IFC_obj_ID"
  Data Type Conversion81/1 -> BusCreator2/39  "RadarCrossSection"
  Data Type Conversion196/1 -> BusCreator1/34  "RFtar_MovingState"
  Ground12/1 -> BusCreator4/110  "IFC_Roaddge01_DxEnd"
  Subsystem73/1(RFtar_Width) -> Data Type Conversion163/1  "RFtar_Width"
  Data Type Conversion245/1 -> BusCreator4/98  "IFC_Line04_LineID"
  Read CM Dict29/1 -> Data Type Conversion216/1
  Data Type Conversion54/1 -> BusCreator4/53  "IFC_Line01_Curv"
  Data Type Conversion255/1 -> BusCreator2/19  "AbsoluteLatAcc"
  Data Type Conversion231/1 -> BusCreator4/85  "IFC_Line03_LineID"
  Read CM Dict12/1 -> Data Type Conversion59/1
  Data Type Conversion251/1 -> BusCreator4/103  "IFC_Line04_LineWidth"
  Subsystem86/1(LBtar_Xpos) -> Data Type Conversion175/1  "LBtar_Xpos"
  Data Type Conversion228/1 -> BusCreator4/82  "IFC_Line03_ExistProb"
  Data Type Conversion69/1 -> BusCreator4/124  "camera_timestamp"
  Data Type Conversion454/1 -> BusCreator/10  "obj_vd_unt"
  Constant13/1 -> Data Type Conversion448/1
  Data Type Conversion452/1 -> BusCreator/8  "lap_is_nstruction_area"
  Constant14/1 -> Data Type Conversion453/1
  Constant20/1 -> Data Type Conversion443/1
  Data Type Conversion443/1 -> BusCreator/1  "LH_Snow_Road_Prob"
  Constant17/1 -> Data Type Conversion455/1
  Constant16/1 -> Data Type Conversion454/1
  Constant18/1 -> Data Type Conversion451/1
  Constant21/1 -> Data Type Conversion444/1
  Data Type Conversion455/1 -> BusCreator/11  "obj_anil"
  Data Type Conversion448/1 -> BusCreator/5  "lap_is_ghway_merge_left"
  Constant12/1 -> Data Type Conversion447/1
  Constant15/1 -> Data Type Conversion442/1
  Constant11/1 -> Data Type Conversion449/1
  Data Type Conversion446/1 -> BusCreator/3  "con_Is_ghspedd_road"
  Data Type Conversion449/1 -> BusCreator/6  "lap_is_ghway_exit_right"
  Data Type Conversion444/1 -> BusCreator/2  "con_Is_ghspedd_road_v"
  Data Type Conversion447/1 -> BusCreator/4  "lap_is_ghway_merge_right"
  Constant10/1 -> Data Type Conversion446/1
  Data Type Conversion442/1 -> BusCreator4/140  "obj_rel_axstddev"
  Constant8/1 -> Data Type Conversion398/1
  Constant19/1 -> Data Type Conversion452/1
  Data Type Conversion398/1 -> BusCreator4/137  "obj_motion"
  Data Type Conversion451/1 -> BusCreator/7  "lap_is_ghway_exit_left"
  Data Type Conversion453/1 -> BusCreator/9  "obj_vruount"
  Ground43/1 -> BusCreator4/138  "obj_lane_Assignmenr"
  Ground44/1 -> BusCreator4/139  "obj_age"
  BusCreator/1 -> To Workspace4/1
  Ground47/1 -> BusCreator4/141  "obj_rel_ax"

== system MIL4L3_SW6_V1_20220211/CarMaker/VehicleControl/SwitchForRealECU_ACC_Brake ==
  In1 : Inport
  Define CM Dict1 : CarMaker4SL/Define CM Dict  xname=User.IO.In.Radar.RealECUSW_ACC  xunit=m/s2  xmono=off  xtype=Double4  xdvaplace=IO_In  xnstates=0  xfirststate=0  xinitial=0
  Define CM Dict2 : CarMaker4SL/Define CM Dict  xname=User.IO.In.Radar.BrakeDecManual  xunit=m/s2  xmono=off  xtype=Double4  xdvaplace=IO_In  xnstates=0  xfirststate=0  xinitial=0
  Define CM Dict3 : CarMaker4SL/Define CM Dict  xname=User.IO.In.Radar.BrakeDecManualSW  xunit=m/s2  xmono=off  xtype=Double4  xdvaplace=IO_In  xnstates=0  xfirststate=0  xinitial=0
  PI Control : Subsystem
  Read CM Dict2 : CarMaker4SL/Read CM Dict  xname=User.IO.In.Radar.BrakeDecManual  xsync=off
  Read CM Dict3 : CarMaker4SL/Read CM Dict  xname=User.IO.In.Radar.BrakeDecManualSW  xsync=off
  Read CM Dict5 : CarMaker4SL/Read CM Dict  xname=User.IO.In.Radar.RealECUSW_ACC  xsync=off
  Switch : Switch  Criteria=u2 > Threshold
  Switch1 : Switch  Criteria=u2 > Threshold
  Out1 : Outport
  wires:
  In1/1 -> Switch/3
  Switch1/1 -> Switch/1
  Read CM Dict2/1 -> Switch1/2, Switch1/1
  Read CM Dict5/1 -> Switch/2
  PI Control/1(Out1) -> Switch1/3
  Switch/1 -> Out1/1

== system MIL4L3_SW6_V1_20220211/CarMaker/VehicleControl/SwitchForRealECU_ACC_Gas ==
  note: Brake first
  In1 : Inport
  Compare To Constant2 : simulink/Logic and Bit Operations/Compare To Constant  relop===  const=1  OutDataTypeStr=boolean
  Constant1 : Constant  Value=0
  Constant3 : Constant  Value=0
  Define CM Dict2 : CarMaker4SL/Define CM Dict  xname=User.IO.In.Radar.GasAxManual  xunit=m/s2  xmono=off  xtype=Double4  xdvaplace=IO_In  xnstates=0  xfirststate=0  xinitial=0
  Define CM Dict3 : CarMaker4SL/Define CM Dict  xname=User.IO.In.AEB_Braking_progress  xmono=off  xtype=Double4  xdvaplace=IO_In  xnstates=0  xfirststate=0  xinitial=0
  Define CM Dict5 : CarMaker4SL/Define CM Dict  xname=User.IO.Out.GasPdlPsn  xunit=m/s2  xmono=off  xtype=Double4  xdvaplace=IO_In  xnstates=0  xfirststate=0  xinitial=0
  PI Control : Subsystem
  Read CM Dict1 : CarMaker4SL/Read CM Dict  xname=User.IO.In.Radar.RealECUSW_ACC  xsync=off
  Read CM Dict2 : CarMaker4SL/Read CM Dict  xname=User.IO.In.Radar.GasAxManual  xsync=off
  Read CM Dict4 : CarMaker4SL/Read CM Dict  xname=User.IO.In.AEB_Braking_progress  xsync=off
  Relational Operator : RelationalOperator  OutDataTypeStr=boolean  RndMeth=Nearest
  Saturation1 : Saturate  UpperLimit=1  LowerLimit=0
  Switch{,1..3} (4 alike) : Switch  Criteria=u2 > Threshold  Threshold=0.5
  Write CM Dict : CarMaker4SL/Write CM Dict  xname=User.IO.Out.GasPdlPsn  xsync=off
  Out1 : Outport
  wires:
  In1/1 -> Switch/3
  Constant3/1 -> Switch1/3
  Compare To Constant2/1 -> Switch1/2
  Switch1/1 -> PI Control/1(In1)
  PI Control/1(Out1) -> Switch/1
  Switch/1 -> Switch3/3, Relational Operator/2
  Read CM Dict2/1 -> Relational Operator/1, Switch3/1
  Relational Operator/1 -> Switch3/2
  [ADAS_TorqueActivReq] -> Compare To Constant2/1
  Read CM Dict1/1 -> Switch/2
  [ACCTqReq] -> Switch1/1
  Switch3/1 -> Switch2/3
  Constant1/1 -> Switch2/1
  Saturation1/1 -> Write CM Dict/1, Out1/1
  Read CM Dict4/1 -> Switch2/2
  Switch2/1 -> Saturation1/1
